simulink model "ISReferenceApplication"  (R2019b)
settings: Solver=VariableStepAuto  StartTime=0.0  StopTime=10.0  RelTol=1e-3
undefined symbols (not defined in the file or in its folder): C_Brake, C_Final, C_Front, C_Middle, C_out_Brake, C_out_Final, C_out_Front, C_out_Middle, Co, Cso, D_out_Brake, D_out_Final, D_out_Front, D_out_Middle, Downshift_Speeds, F, F_Brake, F_Final, F_Front, F_Middle, Fs, G_Brake, G_Final, G_Front, G_Middle, G_sys_Brake, G_sys_Final, G_sys_Front, G_sys_Middle, Gd, Gd_Brake, Gd_Final, Gsd, h, H_Brake, H_Final, H_Front, H_Middle, H_sys_Brake, H_sys_Final, H_sys_Front, H_sys_Middle, Hd, Hd_Brake, Hd_Final, Hsd, JE, JE_Brake, JE_Final, JE_Front, JE_Middle, JEs, JF_part, JF_part_Brake, JF_part_Final, JF_parts, Ld, Ld_Brake, Ld_Final, Ld_Front ... (+21)
libraries: simulink x5, autolibutils x3, sim3dlib x2, vehdynlibviscommon x1
(part 3 of 4)

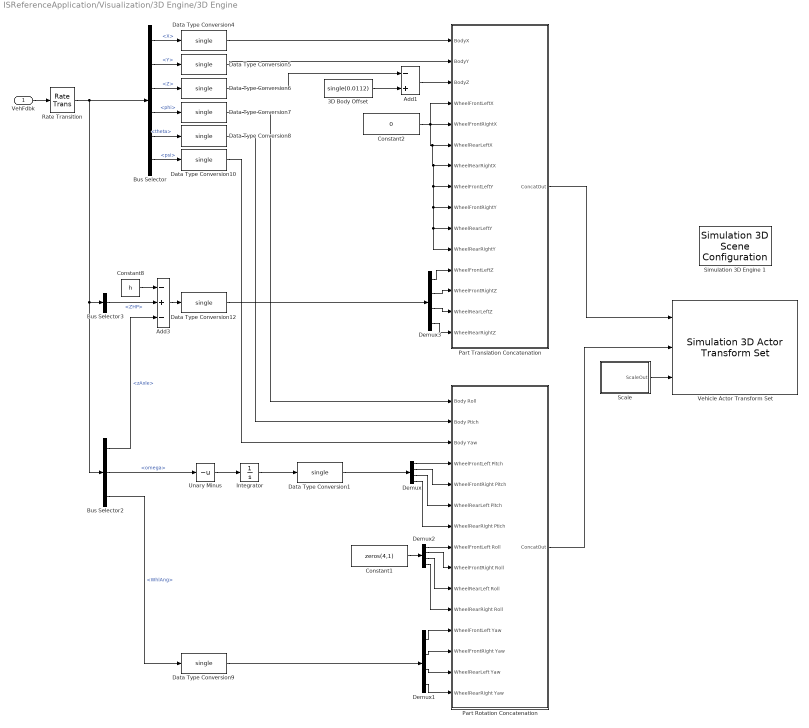
== system ISReferenceApplication/Visualization/3D Engine/3D Engine ==
  VehFdbk : Inport
  3D Body Offset : Constant  Value=single(0.0112)  OutDataTypeStr=single
  Add1 : Sum  Inputs=-+
  Add3 : Sum  Inputs=-+-
  Bus Selector : BusSelector  OutputSignals=Body.X,Body.Y,Body.Z,Body.phi,Body.theta,Body.psi
  Bus Selector2 : BusSelector  OutputSignals=Wheels.zAxle,Wheels.omega,Driveline.WhlAng
  Bus Selector3 : BusSelector  OutputSignals=Body.ZHP
  Constant1 : Constant  Value=zeros(4,1)  OutDataTypeStr=single
  Constant2 : Constant  Value=0  OutDataTypeStr=single
  Constant8 : Constant  Value=h
  Data Type Conversion{1,4..10,12} (9 alike) : DataTypeConversion  OutDataTypeStr=single
  Demux{,1..3} (4 alike) : Demux
  Integrator : Integrator  WrapState=on  WrappedStateUpperValue=2*pi  WrappedStateLowerValue=0  ZeroCross=off
  Part Rotation Concatenation : Subsystem
  Part Translation Concatenation : Subsystem
  Rate Transition : RateTransition  OutPortSampleTime=dt3D
  Scale : Subsystem
  Simulation 3D Engine 1 : sim3dlib/Simulation 3D Scene Configuration  Priority=1  SceneDesc=Straight road  vehTagList={'Scene Origin'}  vehTag=Scene Origin  OpVisEn=off  Ts=dt3D  ProjectFormat=Executable  ProjectName=VehicleSimulation.exe  sensorTag=MainCamera1  sensorId=1  sensorName=MainCamera1  mountLoc=Origin  offsetFlag=off  tmountOffset=[0, 0, 0]  rmountOffset=[0, 0, 0]  HorizontalResolution=1280  VerticalResolution=720  HorizontalFOV=60  mountPoint=[0 0 0]  mountOrientation=[0 0 0]  aMode=aMode  ID=1
      settings: AttributesFormatString=Priority: %<Priority>  SourceProductName=Automated Driving Toolbox  SourceProductBaseCode=DR
  Unary Minus : UnaryMinus
  Vehicle Actor Transform Set : sim3dlib/Simulation 3D Actor Transform Set  ActorTag=SimulinkVehicle1  ActorType=Passenger vehicle  PassVehMesh=Muscle car  VehColor=Red  NumberOfParts=5  CustNumOfParts=3  Translation=[0 0 1; 0 0 0; 0 0 0; 0 0 0; 0 0 0]  Rotation=[0 0 0; 0 0 0; 0 0 0; 0 0 0; 0 0 0]  Scale=[1 1 1; 1 1 1; 1 1 1; 1 1 1; 1 1 1]  Ts=dt3D
      settings: SourceProductName=Automated Driving Toolbox  SourceProductBaseCode=DR
  wires:
  Bus Selector/5 -> Data Type Conversion8/1  "<theta>"
  Bus Selector/6 -> Data Type Conversion10/1  "<psi>"
  Bus Selector/3 -> Data Type Conversion6/1  "<Z>"
  Bus Selector/2 -> Data Type Conversion5/1  "<Y>"
  Bus Selector/1 -> Data Type Conversion4/1  "<X>"
  Data Type Conversion7/1 -> Part Rotation Concatenation/1(Body Roll)
  Data Type Conversion4/1 -> Part Translation Concatenation/1(BodyX)
  Constant2/1 -> Part Translation Concatenation/4(WheelFrontLeftX), Part Translation Concatenation/11(WheelRearRightY), Part Translation Concatenation/10(WheelRearLeftY), Part Translation Concatenation/9(WheelFrontRightY), Part Translation Concatenation/8(WheelFrontLeftY), Part Translation Concatenation/7(WheelRearRightX), Part Translation Concatenation/6(WheelRearLeftX), Part Translation Concatenation/5(WheelFrontRightX)
  Data Type Conversion10/1 -> Part Rotation Concatenation/3(Body Yaw)
  Data Type Conversion5/1 -> Part Translation Concatenation/2(BodyY)
  Data Type Conversion8/1 -> Part Rotation Concatenation/2(Body Ptich)
  Data Type Conversion1/1 -> Demux/1
  Integrator/1 -> Data Type Conversion1/1
  Demux1/2 -> Part Rotation Concatenation/13(WheelFrontRight Yaw)
  Demux1/1 -> Part Rotation Concatenation/12(WheelFrontLeft Yaw)
  Data Type Conversion9/1 -> Demux1/1
  Bus Selector2/2 -> Unary Minus/1  "<omega>"
  Bus Selector2/3 -> Data Type Conversion9/1  "<WhlAng>"
  Demux2/4 -> Part Rotation Concatenation/11(WheelRearRight Roll)
  Demux2/3 -> Part Rotation Concatenation/10(WheelRearLeft Roll)
  Demux2/2 -> Part Rotation Concatenation/9(WheelFrontRight Roll)
  Demux2/1 -> Part Rotation Concatenation/8(WheelFrontLeft Roll)
  Demux1/3 -> Part Rotation Concatenation/14(WheelRearLeft Yaw)
  Demux1/4 -> Part Rotation Concatenation/15(WheelRearRight Yaw)
  3D Body Offset/1 -> Add1/2
  Add1/1 -> Part Translation Concatenation/3(BodyZ)
  VehFdbk/1 -> Rate Transition/1
  Demux3/2 -> Part Translation Concatenation/13(WheelFrontRightZ)
  Demux3/1 -> Part Translation Concatenation/12(WheelFrontLeftZ)
  Demux3/3 -> Part Translation Concatenation/14(WheelRearLeftZ)
  Demux3/4 -> Part Translation Concatenation/15(WheelRearRightZ)
  Data Type Conversion12/1 -> Demux3/1
  Part Translation Concatenation/1(ConcatOut) -> Vehicle Actor Transform Set/1
  Part Rotation Concatenation/1(ConcatOut) -> Vehicle Actor Transform Set/2
  Data Type Conversion6/1 -> Add1/1
  Bus Selector/4 -> Data Type Conversion7/1  "<phi>"
  Constant1/1 -> Demux2/1
  Demux/1 -> Part Rotation Concatenation/4(WheelFrontLeft Pitch)
  Demux/2 -> Part Rotation Concatenation/5(WheelFrontRight Pitch)
  Demux/3 -> Part Rotation Concatenation/6(WheelRearLeft Pitch)
  Demux/4 -> Part Rotation Concatenation/7(WheelRearRight Ptich)
  Scale/1(ScaleOut) -> Vehicle Actor Transform Set/3
  Rate Transition/1 -> Bus Selector2/1, Bus Selector3/1, Bus Selector/1
  Constant8/1 -> Add3/1
  Bus Selector2/1 -> Add3/3  "<zAxle>"
  Add3/1 -> Data Type Conversion12/1
  Bus Selector3/1 -> Add3/2  "<ZHP>"
  Unary Minus/1 -> Integrator/1

== system ISReferenceApplication/Visualization/3D Engine/3D Engine Disabled ==
  VehFdbk : Inport
  Terminator : Terminator
  wires:
  VehFdbk/1 -> Terminator/1

== system ISReferenceApplication/Controllers1/Brake Controller/Brake Pressure Control/Bang Bang ABS ==
  Pref : Inport
  xdot : Inport  Port=2
  <Kappa> : Inport  Port=3
  Abs : Abs
  Add : Sum  Inputs=-+
  Bang-bang controller : Subsystem  mask(Sign){}
      mask help: y = sign(x)
      mask Help: Sign Function:\n\t\t\ty = 1 if x > 0\n\t\t\ty = 0 if x = 0\n\t\t\ty = -1 if x < 0
      mask Display: plot(-50,-50,50,50,[-50,50],[0,0],[0,0],[-50,50],[-40,0],[-30,-30],[0,40],[30,30])
  Compare To Constant : simulink/Logic and Bit Operations/Compare To Constant  relop=>=  const=.2  OutDataTypeStr=boolean
  Compare To Constant1 : simulink/Logic and Bit Operations/Compare To Constant  relop=>=  const=.75  OutDataTypeStr=boolean
  Compare To Constant2 : simulink/Logic and Bit Operations/Compare To Constant  relop=>=  const=.5  OutDataTypeStr=boolean
  Constant : Constant  Value=.25
  Debounce : autolibutils/Debounce  DbcOn_Cnts=.1*.001  DbcOff_Cnts=.1*.001  aMode=aMode
      settings: SourceProductName=Powertrain Blockset  SourceProductBaseCode=PW
  First Order Hold : FirstOrderHold  ErrorTolerance=1
  Gain : Gain  Gain=200
  Logical Operator : Logic  Inputs=3  AllPortsSameDT=off  OutDataTypeStr=boolean
  Rate Transition : RateTransition  Deterministic=off  OutPortSampleTime=.001
  Switch : Switch  Criteria=u2 > Threshold  ZeroCross=off
  PCmd : Outport  VectorParamsAs1DForOutWhenUnconnected=off
  wires:
  Gain/1 -> Switch/1
  Compare To Constant2/1 -> Logical Operator/1
  Abs/1 -> Compare To Constant2/1
  xdot/1 -> Abs/1
  Debounce/1 -> Switch/2
  Compare To Constant1/1 -> Logical Operator/3
  Compare To Constant/1 -> Logical Operator/2
  Logical Operator/1 -> Debounce/1
  Rate Transition/1 -> Compare To Constant/1, Add/1
  Switch/1 -> First Order Hold/1
  Constant/1 -> Add/2  "slip ref"
  Pref/1 -> Compare To Constant1/1, Switch/3  "Pref"
  <Kappa>/1 -> Rate Transition/1
  First Order Hold/1 -> PCmd/1
  Add/1 -> Bang-bang controller/1(in_1)
  Bang-bang controller/1(out_1) -> Gain/1

== system ISReferenceApplication/Controllers1/Brake Controller/Brake Pressure Control/Open Loop ==
  Pref : Inport
  PCmd : Outport  VectorParamsAs1DForOutWhenUnconnected=off
  wires:
  Pref/1 -> PCmd/1  "Reference Slip"

== system ISReferenceApplication/Controllers1/Transmission Controller/TCM/Neutral Select ==
  AccCmd : Inport
  EngSpd : Inport  Port=2
  Constant : Constant  Value=1200
  Constant1 : Constant  Value=1e-6
  Logical Operator : Logic  AllPortsSameDT=off  OutDataTypeStr=boolean
  Relational Operator : RelationalOperator  Operator=<=  OutDataTypeStr=boolean  RndMeth=Simplest
  Relational Operator1 : RelationalOperator  Operator=<=  OutDataTypeStr=boolean  RndMeth=Simplest
  Neutral Select : Outport  VectorParamsAs1DForOutWhenUnconnected=off
  wires:
  Relational Operator/1 -> Logical Operator/2
  Constant/1 -> Relational Operator/2
  Logical Operator/1 -> Neutral Select/1
  Constant1/1 -> Relational Operator1/2
  AccCmd/1 -> Relational Operator1/1
  Relational Operator1/1 -> Logical Operator/1
  EngSpd/1 -> Relational Operator/1

== system ISReferenceApplication/Controllers1/Transmission Controller/TCM/TCM Shift Controller/calc ==
  note: Determine if next gear will be
      | higher or lower than current gear
  gear : Inport
  pedal : Inport  Port=2
  speed : Inport  Port=3
  f : TriggerPort  TriggerType=function-call  VariantControl=Variant  StatesWhenEnabling=reset
      settings: CopyFcn=Stateflow.SLINSF.SimulinkMan.removeBlockPreDeleteFcn  PreDeleteFcn=Stateflow.SLINSF.SimulinkMan.unsafePredeleteFcn
  Add1 : Sum  Inputs=+-
  Add3 : Sum  Inputs=+-
  Add4 : Sum  Inputs=+-
  Calculate Upshift Threshold : Lookup_n-D  BreakpointsForDimension1=Pedal_Positions  BreakpointsForDimension2=1:7  Table=Upshift_Speeds  ExtrapMethod=Clip  UseLastTableValue=on  InternalRulePriority=Speed  RndMeth=Simplest  InputSameDT=on
  Calculate Downshift Threshold : Lookup_n-D  BreakpointsForDimension1=Pedal_Positions  BreakpointsForDimension2=2:8  Table=Downshift_Speeds  ExtrapMethod=Clip  UseLastTableValue=on  InternalRulePriority=Speed  RndMeth=Simplest  InputSameDT=on
  SpdThr : Outport  VectorParamsAs1DForOutWhenUnconnected=off
  wires:
  Add4/1 -> SpdThr/1
  Add3/1 -> Add4/2
  Add1/1 -> Add4/1
  speed/1 -> Add3/1, Add1/2
  Calculate Upshift Threshold/1 -> Add1/1
  Calculate Downshift Threshold/1 -> Add3/2
  gear/1 -> Calculate Upshift Threshold/2, Calculate Downshift Threshold/2
  pedal/1 -> Calculate Upshift Threshold/1, Calculate Downshift Threshold/1

== system ISReferenceApplication/Controllers1/Transmission Controller/TCM/TCM Shift Controller/calc_down ==
  gear : Inport
  pedal : Inport  Port=2
  f : TriggerPort  TriggerType=function-call  VariantControl=Variant  StatesWhenEnabling=reset
      settings: CopyFcn=Stateflow.SLINSF.SimulinkMan.removeBlockPreDeleteFcn  PreDeleteFcn=Stateflow.SLINSF.SimulinkMan.unsafePredeleteFcn
  Calculate Downshift Threshold : Lookup_n-D  BreakpointsForDimension1=Pedal_Positions  BreakpointsForDimension2=2:8  Table=Downshift_Speeds  ExtrapMethod=Clip  UseLastTableValue=on  InternalRulePriority=Speed  RndMeth=Simplest  InputSameDT=on
  down_th : Outport  VectorParamsAs1DForOutWhenUnconnected=off
  wires:
  pedal/1 -> Calculate Downshift Threshold/1
  gear/1 -> Calculate Downshift Threshold/2
  Calculate Downshift Threshold/1 -> down_th/1

== system ISReferenceApplication/Controllers1/Transmission Controller/TCM/TCM Shift Controller/calc_up ==
  gear : Inport
  pedal : Inport  Port=2
  f : TriggerPort  TriggerType=function-call  VariantControl=Variant  StatesWhenEnabling=reset
      settings: CopyFcn=Stateflow.SLINSF.SimulinkMan.removeBlockPreDeleteFcn  PreDeleteFcn=Stateflow.SLINSF.SimulinkMan.unsafePredeleteFcn
  Calculate Upshift Threshold : Lookup_n-D  BreakpointsForDimension1=Pedal_Positions  BreakpointsForDimension2=1:7  Table=Upshift_Speeds  ExtrapMethod=Clip  UseLastTableValue=on  InternalRulePriority=Speed  RndMeth=Simplest  InputSameDT=on
  up_th : Outport  VectorParamsAs1DForOutWhenUnconnected=off
  wires:
  gear/1 -> Calculate Upshift Threshold/2
  pedal/1 -> Calculate Upshift Threshold/1
  Calculate Upshift Threshold/1 -> up_th/1

== system ISReferenceApplication/Visualization/3D Engine/3D Engine/Part Rotation Concatenation ==
  Body Roll : Inport
  Body Ptich : Inport  Port=2
  Body Yaw : Inport  Port=3
  WheelFrontLeft Pitch : Inport  Port=4
  WheelFrontRight Pitch : Inport  Port=5
  WheelRearLeft Pitch : Inport  Port=6
  WheelRearRight Ptich : Inport  Port=7
  WheelFrontLeft Roll : Inport  Port=8
  WheelFrontRight Roll : Inport  Port=9
  WheelRearLeft Roll : Inport  Port=10
  WheelRearRight Roll : Inport  Port=11
  WheelFrontLeft Yaw : Inport  Port=12
  WheelFrontRight Yaw : Inport  Port=13
  WheelRearLeft Yaw : Inport  Port=14
  WheelRearRight Yaw : Inport  Port=15
  AllParts : Concatenate  NumInputs=5  Mode=Multidimensional array
  Body : Concatenate  NumInputs=3  Mode=Multidimensional array  ConcatenateDimension=2
  WheelFrontLeft : Concatenate  NumInputs=3  Mode=Multidimensional array  ConcatenateDimension=2
  WheelFrontRight : Concatenate  NumInputs=3  Mode=Multidimensional array  ConcatenateDimension=2
  WheelRearLeft : Concatenate  NumInputs=3  Mode=Multidimensional array  ConcatenateDimension=2
  WheelRearRight : Concatenate  NumInputs=3  Mode=Multidimensional array  ConcatenateDimension=2
  ConcatOut : Outport  VectorParamsAs1DForOutWhenUnconnected=off
  wires:
  WheelFrontRight Yaw/1 -> WheelFrontRight/3
  WheelRearLeft Pitch/1 -> WheelRearLeft/1
  WheelRearRight/1 -> AllParts/5
  WheelRearLeft Roll/1 -> WheelRearLeft/2
  AllParts/1 -> ConcatOut/1
  WheelRearLeft Yaw/1 -> WheelRearLeft/3
  WheelRearRight Roll/1 -> WheelRearRight/2
  WheelFrontRight Pitch/1 -> WheelFrontRight/1
  WheelFrontRight Roll/1 -> WheelFrontRight/2
  WheelRearRight Yaw/1 -> WheelRearRight/3
  WheelFrontRight/1 -> AllParts/3
  WheelRearLeft/1 -> AllParts/4
  Body/1 -> AllParts/1
  WheelRearRight Ptich/1 -> WheelRearRight/1
  WheelFrontLeft/1 -> AllParts/2
  Body Roll/1 -> Body/2
  WheelFrontLeft Roll/1 -> WheelFrontLeft/2
  WheelFrontLeft Yaw/1 -> WheelFrontLeft/3
  WheelFrontLeft Pitch/1 -> WheelFrontLeft/1
  Body Yaw/1 -> Body/3
  Body Ptich/1 -> Body/1

== system ISReferenceApplication/Visualization/3D Engine/3D Engine/Part Translation Concatenation ==
  BodyX : Inport
  BodyY : Inport  Port=2
  BodyZ : Inport  Port=3
  WheelFrontLeftX : Inport  Port=4
  WheelFrontRightX : Inport  Port=5
  WheelRearLeftX : Inport  Port=6
  WheelRearRightX : Inport  Port=7
  WheelFrontLeftY : Inport  Port=8
  WheelFrontRightY : Inport  Port=9
  WheelRearLeftY : Inport  Port=10
  WheelRearRightY : Inport  Port=11
  WheelFrontLeftZ : Inport  Port=12
  WheelFrontRightZ : Inport  Port=13
  WheelRearLeftZ : Inport  Port=14
  WheelRearRightZ : Inport  Port=15
  AllParts : Concatenate  NumInputs=5  Mode=Multidimensional array
  Body : Concatenate  NumInputs=3  Mode=Multidimensional array  ConcatenateDimension=2
  WheelFrontLeft : Concatenate  NumInputs=3  Mode=Multidimensional array  ConcatenateDimension=2
  WheelFrontRight : Concatenate  NumInputs=3  Mode=Multidimensional array  ConcatenateDimension=2
  WheelRearLeft : Concatenate  NumInputs=3  Mode=Multidimensional array  ConcatenateDimension=2
  WheelRearRight : Concatenate  NumInputs=3  Mode=Multidimensional array  ConcatenateDimension=2
  ConcatOut : Outport  VectorParamsAs1DForOutWhenUnconnected=off
  wires:
  WheelFrontRightZ/1 -> WheelFrontRight/3
  WheelRearLeftX/1 -> WheelRearLeft/1
  WheelRearRight/1 -> AllParts/5
  WheelRearLeftY/1 -> WheelRearLeft/2
  AllParts/1 -> ConcatOut/1
  WheelRearLeftZ/1 -> WheelRearLeft/3
  WheelRearRightY/1 -> WheelRearRight/2
  WheelFrontRightX/1 -> WheelFrontRight/1
  WheelFrontRightY/1 -> WheelFrontRight/2
  WheelRearRightZ/1 -> WheelRearRight/3
  WheelFrontRight/1 -> AllParts/3
  WheelRearLeft/1 -> AllParts/4
  Body/1 -> AllParts/1
  WheelRearRightX/1 -> WheelRearRight/1
  WheelFrontLeft/1 -> AllParts/2
  BodyY/1 -> Body/2
  WheelFrontLeftY/1 -> WheelFrontLeft/2
  WheelFrontLeftZ/1 -> WheelFrontLeft/3
  WheelFrontLeftX/1 -> WheelFrontLeft/1
  BodyZ/1 -> Body/3
  BodyX/1 -> Body/1

== system ISReferenceApplication/Visualization/3D Engine/3D Engine/Scale ==
  Constant{1..12,17,32..33} (15 alike) : Constant  OutDataTypeStr=single
  PartConcatenation : Subsystem
  ScaleOut : Outport  VectorParamsAs1DForOutWhenUnconnected=off
  wires:
  PartConcatenation/1(ConcatOut) -> ScaleOut/1
  Constant12/1 -> PartConcatenation/1(BodyX)
  Constant17/1 -> PartConcatenation/2(BodyY)
  Constant32/1 -> PartConcatenation/3(BodyZ)
  Constant33/1 -> PartConcatenation/4(WheelFrontLeftX)
  Constant1/1 -> PartConcatenation/5(WheelFrontLeftY)
  Constant2/1 -> PartConcatenation/6(WheelFrontLeftZ)
  Constant5/1 -> PartConcatenation/7(WheelFrontRightX)
  Constant3/1 -> PartConcatenation/8(WheelFrontRightY)
  Constant4/1 -> PartConcatenation/9(WheelFrontRightZ)
  Constant8/1 -> PartConcatenation/10(WheelRearLeftX)
  Constant6/1 -> PartConcatenation/11(WheelRearLeftY)
  Constant7/1 -> PartConcatenation/12(WheelRearLeftZ)
  Constant11/1 -> PartConcatenation/13(WheelRearRightX)
  Constant9/1 -> PartConcatenation/14(WheelRearRightY)
  Constant10/1 -> PartConcatenation/15(WheelRearRightZ)

== system ISReferenceApplication/Controllers1/Brake Controller/Brake Pressure Control/Bang Bang ABS/Bang-bang controller ==
  in_1 : Inport
  Constant : Constant  Value=0
  Data Type Conversion1 : DataTypeConversion  OutDataTypeStr=double  SaturateOnIntegerOverflow=on  RndMeth=Zero
  Data Type Conversion2 : DataTypeConversion  OutDataTypeStr=double  SaturateOnIntegerOverflow=on  RndMeth=Zero
  Relational Operator : RelationalOperator  Operator=>  OutDataTypeStr=boolean  RndMeth=Nearest  InputSameDT=on
  Relational Operator1 : RelationalOperator  Operator=<  OutDataTypeStr=boolean  RndMeth=Nearest  InputSameDT=on
  Sum : Sum  Inputs=+-  SaturateOnIntegerOverflow=on  InputSameDT=on  OutDataTypeStr=Inherit: Same as first input
  out_1 : Outport  InitialOutput=0  VectorParamsAs1DForOutWhenUnconnected=off
  wires:
  in_1/1 -> Relational Operator/1, Relational Operator1/1
  Constant/1 -> Relational Operator1/2, Relational Operator/2
  Relational Operator1/1 -> Data Type Conversion2/1
  Relational Operator/1 -> Data Type Conversion1/1
  Sum/1 -> out_1/1
  Data Type Conversion1/1 -> Sum/1
  Data Type Conversion2/1 -> Sum/2

== system ISReferenceApplication/Visualization/3D Engine/3D Engine/Scale/PartConcatenation ==
  BodyX : Inport
  BodyY : Inport  Port=2
  BodyZ : Inport  Port=3
  WheelFrontLeftX : Inport  Port=4
  WheelFrontLeftY : Inport  Port=5
  WheelFrontLeftZ : Inport  Port=6
  WheelFrontRightX : Inport  Port=7
  WheelFrontRightY : Inport  Port=8
  WheelFrontRightZ : Inport  Port=9
  WheelRearLeftX : Inport  Port=10
  WheelRearLeftY : Inport  Port=11
  WheelRearLeftZ : Inport  Port=12
  WheelRearRightX : Inport  Port=13
  WheelRearRightY : Inport  Port=14
  WheelRearRightZ : Inport  Port=15
  AllParts : Concatenate  NumInputs=5  Mode=Multidimensional array
  Body : Concatenate  NumInputs=3  Mode=Multidimensional array  ConcatenateDimension=2
  WheelFrontLeft : Concatenate  NumInputs=3  Mode=Multidimensional array  ConcatenateDimension=2
  WheelFrontRight : Concatenate  NumInputs=3  Mode=Multidimensional array  ConcatenateDimension=2
  WheelRearLeft : Concatenate  NumInputs=3  Mode=Multidimensional array  ConcatenateDimension=2
  WheelRearRight : Concatenate  NumInputs=3  Mode=Multidimensional array  ConcatenateDimension=2
  ConcatOut : Outport  VectorParamsAs1DForOutWhenUnconnected=off
  wires:
  WheelFrontRightZ/1 -> WheelFrontRight/3
  WheelRearLeftX/1 -> WheelRearLeft/1
  WheelRearRight/1 -> AllParts/5
  WheelRearLeftY/1 -> WheelRearLeft/2
  AllParts/1 -> ConcatOut/1
  WheelRearLeftZ/1 -> WheelRearLeft/3
  WheelRearRightY/1 -> WheelRearRight/2
  WheelFrontRightX/1 -> WheelFrontRight/1
  WheelFrontRightY/1 -> WheelFrontRight/2
  WheelRearRightZ/1 -> WheelRearRight/3
  WheelFrontRight/1 -> AllParts/3
  WheelRearLeft/1 -> AllParts/4
  Body/1 -> AllParts/1
  WheelRearRightX/1 -> WheelRearRight/1
  WheelFrontLeft/1 -> AllParts/2
  BodyY/1 -> Body/2
  WheelFrontLeftY/1 -> WheelFrontLeft/2
  WheelFrontLeftZ/1 -> WheelFrontLeft/3
  WheelFrontLeftX/1 -> WheelFrontLeft/1
  BodyZ/1 -> Body/3
  BodyX/1 -> Body/1

== matlab function ISReferenceApplication/Mpc_block/Mpc ==
  data: U_delay input; JE input; JF_part input; Fxh input; M input; Np input; U_min input; U_max input; Heading_updated input; Velocity_updated input; Rs input; Tsim input; Upd_end input; U output; r output; lambda output
function [U, r, lambda] = HQP(U_delay, JE, JF_part, Fxh, M, Np, U_min, U_max, Heading_updated, Velocity_updated, Rs, Tsim,Upd_end)
U = zeros(2,1);
% coder.varsize('Vup', [5 1]);
% disp(sprintf('Simulation time : %2.2f sec',Tsim)) 
% if (Tsim==0)
%     plot(XYplot(:,2),XYplot(:,1));
% end
% if Tsim > 68 %(sec)
%     u1_max =  5/3*pi; u1_min = -5/3*pi;
%     u1_max =  -1; u1_min = -1.05;
%     u2_max =  -0.1; u2_min = -0.12;
%     du1_inc =  0.005*5/3*pi; 
%     du1_dec =  0.005*5/3*pi; 
%     du2_inc =  0.005;
%     du2_dec =  0.005;
% else 

    du1_inc = 1*5/3*pi;
    du1_dec = 1*5/3*pi;
    du2_inc = 1;
    du2_dec = 1;
%     du2_inc = 0.64;
%     du2_dec = 0.64;
% end
% du1_max =  0.1*abs(Fxh(1,:)); 
% du2_max =  0.05*abs(Fxh(1,:)); 
% Y1_min = Rs(1,:) - 2;%V
% Y1_max = Rs(1,:) + 2;%V
% Y2_min = Rs(2,:) - 0.2;%Y
% Y2_max = Rs(2,:) + 0.2;%Y
% 
% Y1_min = -10;%V
% Y2_min = -100;%Y
% Y1_max = 50;%V
% Y2_max = 100;%Y

% Y_max = [];
% Y_min = [];
% for i = 1:Np
%     Y_max = [Y_max;[Y1_max;Y2_max]];
%     Y_min = [Y_min;[Y1_min;Y2_min]];
% end

% U_max = []; U_min = [];
% for i = 1:Np
%     U_max = [U_max; [u1_max; u2_max]];
%     U_min = [U_min; [-u1_min; -u2_min]];
% end

dU_plus = []; dU_minus = [];
for i = 1:Np
    dU_plus = [dU_plus; [U_delay(1) + du1_inc; U_delay(2) + du2_inc]];
    dU_minus = [dU_minus; [-U_delay(1) + du1_dec; -U_delay(2) + du2_dec;]];
end
N = [U_max;
      U_min;
      dU_plus;
      dU_minus;          
     ];
 
% rr_y = [Y_max - Fxh;
%        -Y_min + Fxh;
%        ];

% N = [rr;rr_y];
% if Tsim > 0.1
%     Rs = [];
%     for i = 1:Np
%         Rs = [Rs; Rs_V(i,:); Yup(i,:)];
%     end
% else 
%     Rs = [];
%     for i = 1:Np
%         Rs = [Rs; Rs_V(i,:); Rs_Y(i,:)];
%     end
% end

% Rs = [];
% for i = 1:Np
%     Rs = [Rs; Rs_V(i,:); Rs_heading_angle];
% end
% 

if Tsim > 0 && Tsim < Upd_end
    for i = 1: Np
        Rs(2*i,:) = Heading_updated(i,:);
        Rs(2*i-1,:) = Velocity_updated(i,:);
    end
end


JF = JF_part*(Rs-Fxh);
[u,lambda]= HQP(JE,JF,M,N);
U = u(1:2);

% Extrapolation

% if (Tsim >= Timetochange && Tsim < Timetochange + 0.5)
%     
%     pp = [0 0 1; Ts^2 Ts 1; 4*Ts^2 2*Ts 1];
%     vv = [u3(1,:); u2(1,:); u1(1,:)];
%     abc = inv(pp)*vv;
%     Ue(1,:) = polyval(abc,((Tsim-Timetochange)/Ts+2)*Ts);
%     vv = [u3(2,:); u2(2,:); u1(2,:)];
%     abc = inv(pp)*vv;
%     Ue(2,:) = polyval(abc,((Tsim-Timetochange)/Ts+2)*Ts);
%     U = Ue;
% elseif (Tsim >= Timetochange2 && Tsim < Timetochange2 + 1)
%     
%     pp = [0 0 1; Ts^2 Ts 1; 4*Ts^2 2*Ts 1];
%     vv = [u3(1,:); u2(1,:); u1(1,:)];
%     abc = inv(pp)*vv;
%     Ue(1,:) = polyval(abc,((Tsim-Timetochange2)/Ts+2)*Ts);
%     vv = [u3(2,:); u2(2,:); u1(2,:)];
%     abc = inv(pp)*vv;
%     Ue(2,:) = polyval(abc,((Tsim-Timetochange2)/Ts+2)*Ts);
%     U = Ue;
% else
%     U = un;
% end

% if Tsim <= Timetochange
%     U(1,:) = 1e-9;
% end
r = Rs(1:2,:);
% lambda
end

== stateflow chart ISReferenceApplication/Controllers1/Transmission Controller/TCM/TCM Shift Controller ==
  settings: sampleTime=0.01
  state GearState [parallel]
    settings: executionOrder=1
    state Neutral
      en:
      GearState = 0;
    state G1
      en:
      GearState = 1;
    state G2
      en:
      GearState = 2;
      du:
      [SpdThr] = calc(2,pedal,speed);
    state G3
      en:
      GearState = 3;
      du:
      [SpdThr] = calc(3,pedal,speed);
    state G8
      en:
      GearState = 8;
    state G7
      en:
      GearState = 7;
    state G6
      en:
      GearState = 6;
    state G5
      en:GearState=5;
      du:[SpdThr]=calc(5,pedal,speed);
    state G4
      en:
      GearState = 4;
      du:
      [SpdThr] = calc(4,pedal,speed);
    (default) -> G1
    Neutral -> G1 : [~Neutral]
    G1 -> G2 [order 1] : Up
    G2 -> G3 [order 1] : Up
    G1 -> Neutral [order 2] : [Neutral]
    G2 -> G1 [order 2] : Down
    G3 -> G2 [order 2] : Down
    G3 -> G4 [order 1] : Up
    G4 -> G3 [order 2] : Down
    G7 -> G8 [order 1] : Up
    G5 -> G6 [order 1] : Up
    G6 -> G7 [order 1] : Up
    G4 -> G5 [order 1] : Up
    G5 -> G4 [order 2] : Down
    G6 -> G5 [order 2] : Down
    G7 -> G6 [order 2] : Down
    G8 -> G7 : Down
  state SelectionState [parallel]
    du:[up_th]=calc_up(GearState,pedal);
    du:[down_th]=calc_down(GearState,pedal);
    settings: executionOrder=2
    state SteadyState
      en:
      clutchControl = 0;
    state preDownShifting
    state preUpShifting
    state UpShifting
      en:
      GearState = GearState + 0.5;
    state DownShifting
      en:
      GearState = GearState - 0.5;
    (default) -> SteadyState
    SteadyState -> (junction 62) [order 1] : [speed < down_th && ...
        | GearState >1]
    SteadyState -> (junction 128) [order 2] : [speed > up_th &&...
        | GearState <= 5 && ...
        | floor(GearState) == GearState]
    (junction 62) -> preDownShifting
    (junction 128) -> preUpShifting
    (junction 168) -> SteadyState
    (junction 23) -> SteadyState
    (junction 161) -> SteadyState
    preDownShifting -> (junction 168) [order 2] : [speed >= down_th]
    preUpShifting -> (junction 161) [order 2] : [speed <= up_th]
    preUpShifting -> UpShifting [order 1] : after(0.5,sec)
        | [speed>up_th]
    preDownShifting -> DownShifting [order 1] : after(0.5, sec)
        | [speed < down_th - 2]
    DownShifting -> (junction 23) : {GearState.Down;}
    UpShifting -> (junction 23) : {GearState.Up;}
  state up_th = calc_up(gear,pedal) [function]
  state down_th = calc_down(gear,pedal) [function]
  state SpdThr = calc(gear,pedal,speed) [function]
  data: gear function_input; pedal function_input; up_th function_output; gear function_input; pedal function_input; down_th function_output; gear function_input; pedal function_input; SpdThr function_output; speed function_input; GearState output int8; speed input; pedal input; clutchControl local double; SpdThr local double; Neutral input; up_th local double; down_th local double
  events: Up local EITHER_EDGE_EVENT; Down local EITHER_EDGE_EVENT

== matlab function ISReferenceApplication/MATLAB Function ==
  data: u input; Ac output; Br output
function [Ac, Br] = choose(u)
Ac = 0; Br = 0;
if u > 0 || u == 0
    Ac = u;
else
    Br = abs(u);
end
end

== matlab function ISReferenceApplication/Middle Observer2/Subsystem/Mpc_Simulator_Middle/MATLAB Function ==
  data: Upd_flag input; Timetochange input; Ref output; JE input; U output; M input; Np input; phi input; Qc input; Fxh input; Yup input; Vup input; Rs input; Tsim input; Upd_end input; u input
function [Ref,U] = HQP(Upd_flag, Timetochange, JE,M,Np,phi,Qc,Fxh,Yup,Vup,Rs,Tsim,Upd_end,u)

% if Tsim < 6.27 %(sec)
%     u1_max =  5/3*pi; u1_min = -5/3*pi;
%     u2_max =  0.3; u2_min = -1;
%     du1_inc =  1*5/3*pi; 
%     du1_dec =  1*5/3*pi; 
%     du2_inc =  0.03;
%     du2_dec =  0.03;
% else 
    u1_max =  5/3*pi; u1_min = -5/3*pi;
    u2_max =  1; u2_min = -1;
    du1_inc =  1*5/3*pi;
    du1_dec =  1*5/3*pi;
    du2_inc =  1;
    du2_dec =  1;
% end
% du1_max =  0.1*abs(Fxh(1,:)); 
% du2_max =  0.05*abs(Fxh(1,:)); 
% Y1_min = Rs(1,:) - 2;%V
% Y1_max = Rs(1,:) + 2;%V
% Y2_min = Rs(2,:) - 0.2;%Y
% Y2_max = Rs(2,:) + 0.2;%Y
% 
% Y1_min = -10;%V
% Y2_min = -100;%Y
% Y1_max = 50;%V
% Y2_max = 100;%Y

% Y_max = [];
% Y_min = [];
% for i = 1:Np
%     Y_max = [Y_max;[Y1_max;Y2_max]];
%     Y_min = [Y_min;[Y1_min;Y2_min]];
% end

U_max = []; U_min = [];
for i = 1:Np
    U_max = [U_max; [u1_max; u2_max]];
    U_min = [U_min; [-u1_min; -u2_min]];
end

dU_plus = []; dU_minus = [];
for i = 1:Np
    dU_plus = [dU_plus; [u(1) + du1_inc; u(2) + du2_inc]];
    dU_minus = [dU_minus; [-u(1) + du1_dec; -u(2) + du2_dec;]];
end
rr = [U_max;
      U_min;
      dU_plus;
      dU_minus;          
     ];
 
% rr_y = [Y_max - Fxh;
%        -Y_min + Fxh;
%        ];
N = [];
N = rr; 
% N = [rr;rr_y];
if Tsim > 0 && Tsim < Upd_end
    for i = 1: Np
        Rs(2*i,:) = Yup(i,:);
        Rs(2*i-1,:) = Vup(i,:);
    end

% elseif Tsim >= 65
%     for i = 1: Np
%         Rs(2*i,:) = Yup(i,:);
% %         Rs(2*i-1,:) = Vup(i,:);
%     end
end


JF = -2*phi'*Qc*(Rs-Fxh);
[uc,lambda]= HQP(JE,JF,M,N);
U = uc(1:2);
% if Tsim <= Timetochange
%     U(1,:) = 1e-9;
% end
Ref = Rs(1:2,:);
% lambda
end

== matlab function ISReferenceApplication/Passenger Vehicle/beta ==
  data: xdot input; beta output; ydot input; Velocity output
function [beta, Velocity]  = Velocity(xdot, ydot)
beta = 0; Velocity = 0;
Velocity = sqrt(xdot^2 + ydot^2);

xdot = abs(xdot);

beta = atan2(ydot, xdot);
end

== matlab function ISReferenceApplication/Middle Observer2/Subsystem/Pose updete k/Update ==
  settings: updateMethod=DISCRETE  sampleTime=Ts
  data: Rs_V_now input; Rs_Y_now input; XYline input; XYplot input; XYplot_sim input; Last_XYplot_sim input; Velocity_sim input; Last_Velocity_sim input; Heading_sim input; Last_Heading_sim input; Tsim input; Last_Heading_end input; Velocity_updated output; Heading_updated output [1..5]; Heading_end output
function [Velocity_updated, Heading_updated, Heading_end] = Y_update(Rs_V_now, Rs_Y_now, ...
        XYline, XYplot, XYplot_sim, Last_XYplot_sim, Velocity_sim, Last_Velocity_sim, Heading_sim, Last_Heading_sim, ... 
    Tsim, Last_Heading_end)
    disp(sprintf('Simulation time : %2.1f sec',Tsim)) 
    Np = 5; Ts = 0.1;
    Heading_updated = zeros(Np,1); Velocity_updated = zeros(Np,1);Heading_end = 0;
    coder.extrinsic('intersections');
    coder.extrinsic('P2YV');
%     coder.varsize('Velocity_updated_tmp',[5 1]);
%     coder.varsize('Heading_updated_tmp',[5 1]);
     if Tsim == 0 
        plot(XYline(:,2),XYline(:,1),'black');
    end
   

%%Create half-circle    

    N = 30;
    theta = zeros(Np-1,N+1); Veh_circle = zeros(N+1,(Np-1)*2); 
    xp = zeros(1,N+1); yp = zeros(1,N+1); X = [];  Y = []; X_tmp = 0; Y_tmp = 0;
    lookahead = zeros(Np-1,1);
    
    XYplot_sim_tmp = XYplot_sim;    

%     if Velocity_sim > 0.5
        Velocity_ahead = [Velocity_sim; Rs_V_now(2:Np-1,:)];
%     else
%         Velocity_ahead = Rs_V_now;
%     end

    lookahead = Velocity_ahead*Ts;
    Headngahead = [Heading_sim; Rs_Y_now(2:Np-1,:)];
%     lookahead = [1; 1.5; 2; 2.5; 3];
        
    for j = 1:Np-1        
        theta = Headngahead(j,:)-pi/4 : pi/2/N : Headngahead(j,:)+pi/4;
        xp = lookahead(j,:)*cos(theta) + XYplot_sim_tmp(1,:)*ones(1,length(theta));
        yp = lookahead(j,:)*sin(theta) + XYplot_sim_tmp(2,:)*ones(1,length(theta));
        Veh_circle(:,2*j-1:2*j) = [xp' yp'];
       
    %Find the intersection    
         
        [X_tmp, Y_tmp] = intersections(XYplot(:,1), XYplot(:,2), Veh_circle(:,2*j-1), Veh_circle(:,2*j),0); 
        
        if X_tmp == 0 && Y_tmp == 0
%             X = X_tmp(1:j-1,:);
%             Y = Y_tmp(1:j-1,:);
            break;
        end

        X = [X; X_tmp];
        Y = [Y; Y_tmp];   
        XYplot_sim_tmp = [X_tmp; Y_tmp];
        
    end 
    
%%Obtain predict Velocity and Heading angle
   
  
    
    X = [Last_XYplot_sim(1,:); XYplot_sim(1,:); X];
    Y = [Last_XYplot_sim(2,:); XYplot_sim(2,:); Y];
    Vx0 = Last_Velocity_sim*cos(Last_Heading_sim);
    Vy0 = Last_Velocity_sim*sin(Last_Heading_sim);
    Yaw0 = Last_Heading_sim;
     
    T_sample = []; 
    for j = 1:length(X)
        T_sample = [T_sample; Tsim+(j-1)*Ts];
    end
    
   [Velocity_updated, Heading_updated] = P2YV(0, T_sample , X , Y , Vx0 , Vy0 , Yaw0, Np, Last_Heading_end );
   Heading_end = Heading_updated(end,:);

%     Heading_tmp_end = atan2(XYplot(end,2)-XYplot_sim(2,:), XYplot(end,1)-XYplot_sim(1,:));
% 
%     if  ((Heading_tmp_end - Heading_tmp_end_delay) < -5/3*pi) % Angle compensation
%         Heading_flag_end = Heading_flag_end + 1;
%     elseif ((Heading_tmp_end - Heading_tmp_end_delay) > 5/3*pi)
%         Heading_flag_end = Heading_flag_end - 1;
%     end
%     
%     if flag == 1
%         Heading_updated(1:end) = Heading_tmp_end + Heading_flag_end*2*pi;
%     end
%     if Tsim == 1.5
%         figure();
%         plot(XYplot(:,2),XYplot(:,1),'black-');
%         hold on;
%         plot(XYplot_sim(2,:),XYplot_sim(1,:),'b o');
%         plot(Veh_circle(:,2), Veh_circle(:,1),'b-');
%         plot(Veh_circle(:,4), Veh_circle(:,3),'b-');
%         plot(Veh_circle(:,6), Veh_circle(:,5),'b-');
%         plot(Veh_circle(:,8), Veh_circle(:,7),'b-');
%         plot(Veh_circle(:,10), Veh_circle(:,9),'b-');
%         plot(Y, X,'r x');
%     end

end

== matlab function ISReferenceApplication/YV_update_Np/MATLAB Function2 ==
  data: XY_ref input; Velocity_updated output; XYplot_sim input; Velocity_sim input; Yaw_sim input; Tsim input; Heading_updated output
function [Velocity_updated, Heading_updated] = VY_update(XY_ref, XYplot_sim, Velocity_sim, Yaw_sim, Tsim)
    disp(sprintf('Simulation time : %2.1f sec',Tsim)) 
 Ts = 0.1;
 Np = 6;
 Heading_updated = zeros(Np,1); Velocity_updated = zeros(Np,1);
coder.extrinsic('P2YV');

T_sample = []; 
for j = 1:Np+1
    T_sample = [T_sample; Tsim+(j-1)*Ts];
end
X = [];
for i = 1:Np
    X = [X; XY_ref(2*i-1,:)];
end
Y = [];
for i = 1:Np
    Y = [Y; XY_ref(2*i,:)];
end

X = [XYplot_sim(1,:); X];
Y = [XYplot_sim(2,:); Y];   
Vx0 = Velocity_sim*cos(Yaw_sim);
Vy0 = Velocity_sim*sin(Yaw_sim);
Yaw0 = Yaw_sim;

[Velocity_updated, Heading_updated] = P2YV(0,0, T_sample , X , Y , Vx0 , Vy0 , Yaw0, Np, 0, 0 );

end

== matlab function ISReferenceApplication/Middle Observer2/Subsystem/VH2P/YV2P ==
  data: Velocity input; Yaw input; LastVelocity input; LastYaw input; Tsim input; LastTsim input; Lastpostion input; Position output
function Position  = YV2P(Velocity, Yaw,  LastVelocity, LastYaw, Tsim, LastTsim, Lastpostion)
if Tsim >= 0.1
    Position = zeros(2,1);
    X0 = Lastpostion(1,:); Y0 = Lastpostion(2,:);
    Vx = [LastVelocity*cos(LastYaw); Velocity*cos(Yaw)];
    Vy = [LastVelocity*sin(LastYaw); Velocity*sin(Yaw)];
    Yaw_sim = [LastYaw; Yaw];
    T_sample =[LastTsim; Tsim];
    [ X_tmp, Y_tmp] = YV2P( T_sample, X0, Y0, Vx, Vy, Yaw_sim, zeros(2,1) );
    Position = [X_tmp(end,:); Y_tmp(end,:)];
else
    Position = [0; 0];
end

end

== matlab function ISReferenceApplication/Middle Observer2/Subsystem/YV_update_Np/MATLAB Function2 ==
  data: XY_ref input; Velocity_updated output; XY_sim input; LastXY_sim input; Velocity_sim input; LastVelocity_sim input; Yaw_sim input; LastYaw_sim input; Tsim input; Heading_updated output
function [Velocity_updated, Heading_updated] = VY_update(XY_ref, XY_sim, LastXY_sim, Velocity_sim, LastVelocity_sim, Yaw_sim, LastYaw_sim, Tsim)
    disp(sprintf('Simulation time : %2.1f sec',Tsim)) 
 Ts = 0.1;
%  Np = 6;
 Np = 6;
 Heading_updated = zeros(Np,1); Velocity_updated = zeros(Np,1);
coder.extrinsic('P2YV');
% T_sample = [Tsim-0.01; Tsim; Tsim+0.01];
% X = [LastXY_sim(1); XY_sim(1); XY_ref(1,:)];
% Y = [LastXY_sim(2); XY_sim(2); XY_ref(2,:)];

% T_sample = [Tsim-0.01; Tsim; Tsim+0.01; Tsim+0.02];
% X = [LastXY_sim(1); XY_sim(1); XY_ref(1,:); XY_ref(3,:)];
% Y = [LastXY_sim(2); XY_sim(2); XY_ref(2,:); XY_ref(4,:)];

T_sample = []; 
for j = 1:Np+1
    T_sample = [T_sample; Tsim+(j-1)*Ts];
end
X = [];
for i = 1:Np
    X = [X; XY_ref(2*i-1,:)];
end
Y = [];
for i = 1:Np
    Y = [Y; XY_ref(2*i,:)];
end

X = [XY_sim(1,:); X];
Y = [XY_sim(2,:); Y];   
Vx0 = Velocity_sim*cos(Yaw_sim);
Vy0 = Velocity_sim*sin(Yaw_sim);
Yaw0 = Yaw_sim;

[Velocity_updated, Heading_updated] = P2YV(0,0, T_sample , X , Y , Vx0 , Vy0 , Yaw0, Np, 0, 0 );

end

== matlab function ISReferenceApplication/Final Observer2/MATLAB Function1 ==
  data: select_model input; tri output
function tri = trigger(select_model)
tri = 0;
if select_model == 3%% || select_model ==3
    tri=1;
else
    tri=0;
end
end

== matlab function ISReferenceApplication/Middle Observer2/MATLAB Function1 ==
  data: select_model input; tri output
function tri = trigger(select_model)
tri = 0;
if select_model == 1
    tri=1;
else
    tri=0;
end
end

== matlab function ISReferenceApplication/Middle Observer3/Subsystem/Mpc_Simulator_Middle/MATLAB Function ==
  data: Upd_flag input; Timetochange input; Ref output; JE input; U output; M input; Np input; phi input; Qc input; Fxh input; Yup input; Vup input; Rs input; Rs_V input; Tsim input; Upd_end input; u input
function [Ref,U] = HQP(Upd_flag, Timetochange, JE,M,Np,phi,Qc,Fxh,Yup,Vup,Rs,Rs_V,Tsim,Upd_end,u)

% if Tsim < 6.27 %(sec)
%     u1_max =  5/3*pi; u1_min = -5/3*pi;
%     u2_max =  0.3; u2_min = -1;
%     du1_inc =  1*5/3*pi; 
%     du1_dec =  1*5/3*pi; 
%     du2_inc =  0.03;
%     du2_dec =  0.03;
% else 
    u1_max =  5/3*pi; u1_min = -5/3*pi;
    u2_max =  1; u2_min = -1;
    du1_inc =  1*5/3*pi;
    du1_dec =  1*5/3*pi;
    du2_inc =  1;
    du2_dec =  1;
% end
% du1_max =  0.1*abs(Fxh(1,:)); 
% du2_max =  0.05*abs(Fxh(1,:)); 
% Y1_min = Rs(1,:) - 2;%V
% Y1_max = Rs(1,:) + 2;%V
% Y2_min = Rs(2,:) - 0.2;%Y
% Y2_max = Rs(2,:) + 0.2;%Y
% 
% Y1_min = -10;%V
% Y2_min = -100;%Y
% Y1_max = 50;%V
% Y2_max = 100;%Y

% Y_max = [];
% Y_min = [];
% for i = 1:Np
%     Y_max = [Y_max;[Y1_max;Y2_max]];
%     Y_min = [Y_min;[Y1_min;Y2_min]];
% end

U_max = []; U_min = [];
for i = 1:Np
    U_max = [U_max; [u1_max; u2_max]];
    U_min = [U_min; [-u1_min; -u2_min]];
end

dU_plus = []; dU_minus = [];
for i = 1:Np
    dU_plus = [dU_plus; [u(1) + du1_inc; u(2) + du2_inc]];
    dU_minus = [dU_minus; [-u(1) + du1_dec; -u(2) + du2_dec;]];
end
rr = [U_max;
      U_min;
      dU_plus;
      dU_minus;          
     ];
 
% rr_y = [Y_max - Fxh;
%        -Y_min + Fxh;
%        ];
N = [];
N = rr; 
% N = [rr;rr_y];
if Tsim > 0 && Tsim < Upd_end
    for i = 1: Np
        Rs(2*i,:) = Yup(i,:);
        Rs(2*i-1,:) = Vup(i,:);
    end

% elseif Tsim >= 65
%     for i = 1: Np
%         Rs(2*i,:) = Yup(i,:);
% %         Rs(2*i-1,:) = Vup(i,:);
%     end
end


JF = -2*phi'*Qc*(Rs-Fxh);
[uc,lambda]= HQP(JE,JF,M,N);
U = uc(1:2);
% if Tsim <= Timetochange
%     U(1,:) = 1e-9;
% end
Ref = Rs(1:2,:);
% lambda
end

== matlab function ISReferenceApplication/Middle Observer3/Subsystem/Pose updete k/Update ==
  settings: updateMethod=DISCRETE  sampleTime=Ts
  data: Rs_V_now input; Rs_Y_now input; XYline input; XYplot input; XYplot_sim input; Last_XYplot_sim input; Velocity_sim input; Last_Velocity_sim input; Heading_sim input; Last_Heading_sim input; Tsim input; Last_Heading_end input; Velocity_updated output; Heading_updated output [1..5]; Heading_end output
function [Velocity_updated, Heading_updated, Heading_end] = Y_update(Rs_V_now, Rs_Y_now, ...
        XYline, XYplot, XYplot_sim, Last_XYplot_sim, Velocity_sim, Last_Velocity_sim, Heading_sim, Last_Heading_sim, ... 
    Tsim, Last_Heading_end)
    disp(sprintf('Simulation time : %2.1f sec',Tsim)) 
    Np = 5; Ts = 0.1;
    Heading_updated = zeros(Np,1); Velocity_updated = zeros(Np,1);Heading_end = 0;
    coder.extrinsic('intersections');
    coder.extrinsic('P2YV');
%     coder.varsize('Velocity_updated_tmp',[5 1]);
%     coder.varsize('Heading_updated_tmp',[5 1]);
     if Tsim == 0 
        plot(XYline(:,2),XYline(:,1),'black');
    end
   

%%Create half-circle    

    N = 30;
    theta = zeros(Np-1,N+1); Veh_circle = zeros(N+1,(Np-1)*2); 
    xp = zeros(1,N+1); yp = zeros(1,N+1); X = [];  Y = []; X_tmp = 0; Y_tmp = 0;
    lookahead = zeros(Np-1,1);
    
    XYplot_sim_tmp = XYplot_sim;    

%     if Velocity_sim > 0.5
        Velocity_ahead = [Velocity_sim; Rs_V_now(2:Np-1,:)];
%     else
%         Velocity_ahead = Rs_V_now;
%     end

    lookahead = Velocity_ahead*Ts;
    Headngahead = [Heading_sim; Rs_Y_now(2:Np-1,:)];
%     lookahead = [1; 1.5; 2; 2.5; 3];
        
    for j = 1:Np-1        
        theta = Headngahead(j,:)-pi/4 : pi/2/N : Headngahead(j,:)+pi/4;
        xp = lookahead(j,:)*cos(theta) + XYplot_sim_tmp(1,:)*ones(1,length(theta));
        yp = lookahead(j,:)*sin(theta) + XYplot_sim_tmp(2,:)*ones(1,length(theta));
        Veh_circle(:,2*j-1:2*j) = [xp' yp'];
       
    %Find the intersection    
         
        [X_tmp, Y_tmp] = intersections(XYplot(:,1), XYplot(:,2), Veh_circle(:,2*j-1), Veh_circle(:,2*j),0); 
        
        if X_tmp == 0 && Y_tmp == 0
%             X = X_tmp(1:j-1,:);
%             Y = Y_tmp(1:j-1,:);
            break;
        end

        X = [X; X_tmp];
        Y = [Y; Y_tmp];   
        XYplot_sim_tmp = [X_tmp; Y_tmp];
        
    end 
    
%%Obtain predict Velocity and Heading angle
   
  
    
    X = [Last_XYplot_sim(1,:); XYplot_sim(1,:); X];
    Y = [Last_XYplot_sim(2,:); XYplot_sim(2,:); Y];
    Vx0 = Last_Velocity_sim*cos(Last_Heading_sim);
    Vy0 = Last_Velocity_sim*sin(Last_Heading_sim);
    Yaw0 = Last_Heading_sim;
     
    T_sample = []; 
    for j = 1:length(X)
        T_sample = [T_sample; Tsim+(j-1)*Ts];
    end
    
   [Velocity_updated, Heading_updated] = P2YV(0, T_sample , X , Y , Vx0 , Vy0 , Yaw0, Np, Last_Heading_end );
   Heading_end = Heading_updated(end,:);

%     Heading_tmp_end = atan2(XYplot(end,2)-XYplot_sim(2,:), XYplot(end,1)-XYplot_sim(1,:));
% 
%     if  ((Heading_tmp_end - Heading_tmp_end_delay) < -5/3*pi) % Angle compensation
%         Heading_flag_end = Heading_flag_end + 1;
%     elseif ((Heading_tmp_end - Heading_tmp_end_delay) > 5/3*pi)
%         Heading_flag_end = Heading_flag_end - 1;
%     end
%     
%     if flag == 1
%         Heading_updated(1:end) = Heading_tmp_end + Heading_flag_end*2*pi;
%     end
%     if Tsim == 1.5
%         figure();
%         plot(XYplot(:,2),XYplot(:,1),'black-');
%         hold on;
%         plot(XYplot_sim(2,:),XYplot_sim(1,:),'b o');
%         plot(Veh_circle(:,2), Veh_circle(:,1),'b-');
%         plot(Veh_circle(:,4), Veh_circle(:,3),'b-');
%         plot(Veh_circle(:,6), Veh_circle(:,5),'b-');
%         plot(Veh_circle(:,8), Veh_circle(:,7),'b-');
%         plot(Veh_circle(:,10), Veh_circle(:,9),'b-');
%         plot(Y, X,'r x');
%     end

end

== matlab function ISReferenceApplication/Middle Observer3/Subsystem/VH2P/YV2P ==
  data: Velocity input; Yaw input; LastVelocity input; LastYaw input; Tsim input; LastTsim input; Lastpostion input; Position output
function Position  = YV2P(Velocity, Yaw,  LastVelocity, LastYaw, Tsim, LastTsim, Lastpostion)
if Tsim >= 0.1
    Position = zeros(2,1);
    X0 = Lastpostion(1,:); Y0 = Lastpostion(2,:);
    Vx = [LastVelocity*cos(LastYaw); Velocity*cos(Yaw)];
    Vy = [LastVelocity*sin(LastYaw); Velocity*sin(Yaw)];
    Yaw_sim = [LastYaw; Yaw];
    T_sample =[LastTsim; Tsim];
    [ X_tmp, Y_tmp] = YV2P( T_sample, X0, Y0, Vx, Vy, Yaw_sim, zeros(2,1) );
    Position = [X_tmp(end,:); Y_tmp(end,:)];
else
    Position = [0; 0];
end

end

== matlab function ISReferenceApplication/Middle Observer3/Subsystem/YV_update_Np/MATLAB Function2 ==
  data: XY_ref input; Velocity_updated output; XY_sim input; LastXY_sim input; Velocity_sim input; LastVelocity_sim input; Yaw_sim input; LastYaw_sim input; Tsim input; Heading_updated output
function [Velocity_updated, Heading_updated] = VY_update(XY_ref, XY_sim, LastXY_sim, Velocity_sim, LastVelocity_sim, Yaw_sim, LastYaw_sim, Tsim)
    disp(sprintf('Simulation time : %2.1f sec',Tsim)) 
 Ts = 0.1;
%  Np = 6;
 Np = 6;
 Heading_updated = zeros(Np,1); Velocity_updated = zeros(Np,1);
coder.extrinsic('P2YV');
% T_sample = [Tsim-0.01; Tsim; Tsim+0.01];
% X = [LastXY_sim(1); XY_sim(1); XY_ref(1,:)];
% Y = [LastXY_sim(2); XY_sim(2); XY_ref(2,:)];

% T_sample = [Tsim-0.01; Tsim; Tsim+0.01; Tsim+0.02];
% X = [LastXY_sim(1); XY_sim(1); XY_ref(1,:); XY_ref(3,:)];
% Y = [LastXY_sim(2); XY_sim(2); XY_ref(2,:); XY_ref(4,:)];

T_sample = []; 
for j = 1:Np+1
    T_sample = [T_sample; Tsim+(j-1)*Ts];
end
X = [];
for i = 1:Np
    X = [X; XY_ref(2*i-1,:)];
end
Y = [];
for i = 1:Np
    Y = [Y; XY_ref(2*i,:)];
end

X = [XY_sim(1,:); X];
Y = [XY_sim(2,:); Y];   
Vx0 = Velocity_sim*cos(Yaw_sim);
Vy0 = Velocity_sim*sin(Yaw_sim);
Yaw0 = Yaw_sim;

[Velocity_updated, Heading_updated] = P2YV(0,0, T_sample , X , Y , Vx0 , Vy0 , Yaw0, Np, 0, 0 );

end

== matlab function ISReferenceApplication/Final Observer2/Subsystem/MATLAB Function1 ==
  data: select_model input; tri output
function tri = trigger(select_model)
tri = 0;
if  select_model ==3
    tri=1;
else
    tri=0;
end
end

== matlab function ISReferenceApplication/Final Observer2/Subsystem/Mpc_Simulator_Final/MATLAB Function ==
  data: Upd_flag input; Timetochange input; Ref output; JE input; U output; M input; Np input; phi input; Qc input; Fxh input; Yup input; Vup input; Rs input; Tsim input; Upd_end input; u input
function [Ref,U] = HQP(Upd_flag, Timetochange,JE,M,Np,phi,Qc,Fxh,Yup,Vup,Rs,Tsim,Upd_end,u)

% if Tsim < 6.27 %(sec)
%     u1_max =  5/3*pi; u1_min = -5/3*pi;
%     u2_max =  0.3; u2_min = -1;
%     du1_inc =  1*5/3*pi; 
%     du1_dec =  1*5/3*pi; 
%     du2_inc =  0.03;
%     du2_dec =  0.03;
% else 
    u1_max =  5/3*pi; u1_min = -5/3*pi;
    u2_max =  1; u2_min = -1;
    du1_inc =  1*5/3*pi;
    du1_dec =  1*5/3*pi;
    du2_inc =  1;
    du2_dec =  1;
% end
% du1_max =  0.1*abs(Fxh(1,:)); 
% du2_max =  0.05*abs(Fxh(1,:)); 
% Y1_min = Rs(1,:) - 2;%V
% Y1_max = Rs(1,:) + 2;%V
% Y2_min = Rs(2,:) - 0.2;%Y
% Y2_max = Rs(2,:) + 0.2;%Y
% 
% Y1_min = -10;%V
% Y2_min = -100;%Y
% Y1_max = 50;%V
% Y2_max = 100;%Y

% Y_max = [];
% Y_min = [];
% for i = 1:Np
%     Y_max = [Y_max;[Y1_max;Y2_max]];
%     Y_min = [Y_min;[Y1_min;Y2_min]];
% end

U_max = []; U_min = [];
for i = 1:Np
    U_max = [U_max; [u1_max; u2_max]];
    U_min = [U_min; [-u1_min; -u2_min]];
end

dU_plus = []; dU_minus = [];
for i = 1:Np
    dU_plus = [dU_plus; [u(1) + du1_inc; u(2) + du2_inc]];
    dU_minus = [dU_minus; [-u(1) + du1_dec; -u(2) + du2_dec;]];
end
rr = [U_max;
      U_min;
      dU_plus;
      dU_minus;          
     ];
 
% rr_y = [Y_max - Fxh;
%        -Y_min + Fxh;
%        ];
N = [];
N = rr; 
% N = [rr;rr_y];


if Tsim > 0 && Tsim < Upd_end
    for i = 1: Np
        Rs(2*i,:) = Yup(i,:);
        Rs(2*i-1,:) = Vup(i,:);
    end
% elseif Tsim >= 65
%     for i = 1: Np
%         Rs(2*i,:) = Yup(i,:);
% %         Rs(2*i-1,:) = Vup(i,:);
%     end
end


JF = -2*phi'*Qc*(Rs-Fxh);
[uc,lambda]= HQP(JE,JF,M,N);
U = uc(1:2);
% if Tsim <= Timetochange
%     U(1,:) = 1e-9;
% end
Ref = Rs(1:2,:);
% lambda
end
